simulink model "Project_5_lin_s"  (Simulink 8.4)
settings: Solver=ode5  StartTime=0.0  StopTime=10.0  FixedStep=0.01  RelTol=1e-3
undefined symbols (not defined in the file or in its folder): A, B, C, D, x0
settings Model: Creator=cmc4177  LastModifiedBy=cmc4177
settings DataIOCC: SignalLoggingSaveFormat=Dataset
settings OptimizationCC: ExpressionDepthLimit=128
settings DebuggingCC: UnderspecifiedInitializationDetection=Simplified  MergeDetectMultiDrivingBlocksExec=error  FcnCallInpInsideContextMsg=EnableAllAsError  StateNameClashWarn=none
settings GRTTargetCC: CombineOutputUpdateFcns=on  GRTInterface=off

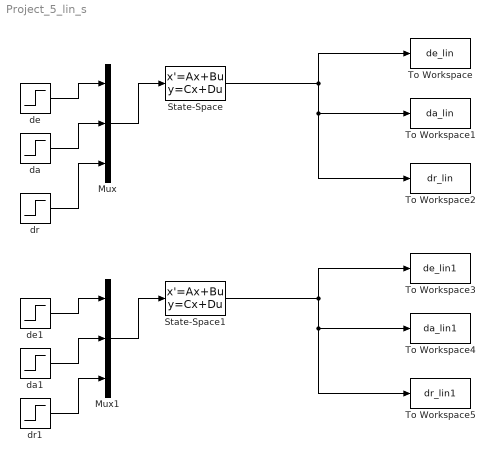
== system Project_5_lin_s ==
  Mux : Mux  Inputs=3
  Mux1 : Mux  Inputs=3
  State-Space : StateSpace  A=A  B=B  C=C  D=D  X0=x0
  State-Space1 : StateSpace  A=A  B=B  C=C  D=D  X0=x0
  To Workspace : ToWorkspace  VariableName=de_lin  SampleTime=-1
  To Workspace1 : ToWorkspace  VariableName=da_lin  SampleTime=-1
  To Workspace2 : ToWorkspace  VariableName=dr_lin  SampleTime=-1
  To Workspace3 : ToWorkspace  VariableName=de_lin1  SampleTime=-1
  To Workspace4 : ToWorkspace  VariableName=da_lin1  SampleTime=-1
  To Workspace5 : ToWorkspace  VariableName=dr_lin1  SampleTime=-1
  da : Step  After=0  SampleTime=0
  da1 : Step  After=-0.5  SampleTime=0
  de : Step  After=-0.5  SampleTime=0
  de1 : Step  After=0  SampleTime=0
  dr : Step  After=0  SampleTime=0
  dr1 : Step  After=0  SampleTime=0
  wires:
  State-Space/1 -> To Workspace/1, To Workspace2/1, To Workspace1/1
  Mux/1 -> State-Space/1
  de/1 -> Mux/1
  da/1 -> Mux/2
  dr/1 -> Mux/3
  State-Space1/1 -> To Workspace4/1, To Workspace5/1, To Workspace3/1
  Mux1/1 -> State-Space1/1
  de1/1 -> Mux1/1
  da1/1 -> Mux1/2
  dr1/1 -> Mux1/3
